simulink model "spi"  (Simulink 6.6)
settings: Solver=ode45  StartTime=0.0  StopTime=2000  RelTol=1e-3
libraries: xbsIndex_r4 x15, xps_library x1
settings Model: Creator=user  LastModifiedBy=SHL
settings GRTTargetCC: TargetFcnLib=ansi_tfl_table_tmw.mat

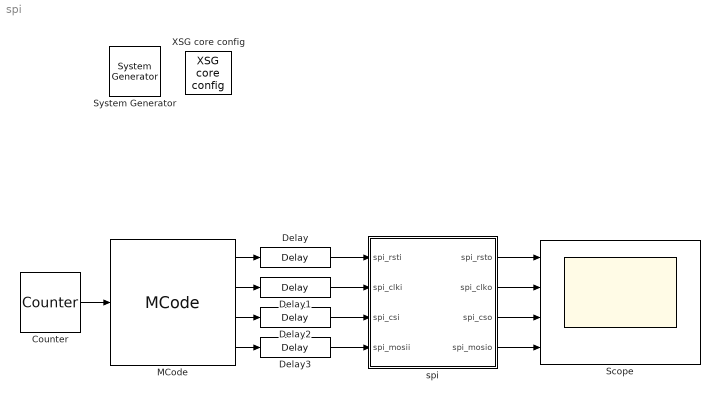
== system spi ==
  " System Generator" : xbsIndex_r4/ System Generator  Tag=genX  SystemSampleTime=-1  xilinxfamily=virtex5  part=xc5vsx95t  speed=-1  package=ff1136  synthesis_tool=XST  clock_wrapper=Clock Enables  directory=./spi/sysgen  testbench=off  simulink_period=1  sysclk_period=10  dcm_input_clock_period=100  incr_netlist=off  trim_vbits=Everywhere in SubSystem  dbl_ovrd=According to Block Masks  core_generation=According to Block Masks  run_coregen=off  deprecated_control=off  eval_field=0  block_type=sysgen
      settings: block_version=10.1.3
  Counter : xbsIndex_r4/Counter  cnt_type=Free Running  cnt_to=Inf  operation=Up  start_count=0  cnt_by_val=1  arith_type=Unsigned  n_bits=4  bin_pt=0  load_pin=off  rst=off  en=off  explicit_period=on  period=1  dbl_ovrd=off  use_behavioral_HDL=off  use_rpm=off  implementation=Fabric  block_type=counter
  Delay{,1..3} (4 alike) : xbsIndex_r4/Delay  en=off  latency=1  dbl_ovrd=off  reg_retiming=on  block_type=delay
  MCode : xbsIndex_r4/MCode  mfname=spi_ctrl  explicit_period=off  period=1  inputsTable={'boundInpExpr'=>[''],'inputs'=>['clk_in']}  outputsTable={'outputs'=>['spi_rst','spi_clk','spi_cs','spi_mosi'],'suppressOut'=>['off','off','off','off']}  dbl_ovrd=off  enable_stdout=off  enable_debug=off  suppress_output=1  defparams={}  hide_port_list={}  block_type=mcode
      settings: block_version=10.1.3
  Scope : Scope  NumInputPorts=4
      settings: TickLabels=on  YMin=-1~-1~-1~-1  YMax=2~2~2~2
  XSG core config : xps_library/XSG core config  Tag=xps:xsg  SystemSampleTime=-1  hw_sys=ROACH:sx95t  ibob_linux=off  clk_src=sys_clk  iBOB_clk_src=sys_clk  BEE2_ctrl_clk_src=sys_clk  BEE2_usr_clk_src=sys_clk  ROACH_clk_src=sys_clk  CORR_clk_src=sys_clk  gpio_clk_io_group=iBOB:sma  gpio_clk_bit_index=0  clk_rate=100  sample_period=1  synthesis_tool=XST  mpc_type=powerpc440_ext
  spi : Subsystem  Tag=xps:spi  AncestorBlock=xps_library/gpio
  wires:
  spi/3(spi_cso) -> Scope/3
  spi/4(spi_mosio) -> Scope/4
  Delay2/1 -> spi/3(spi_csi)
  Delay3/1 -> spi/4(spi_mosii)
  Counter/1 -> MCode/1
  MCode/1 -> Delay/1
  MCode/2 -> Delay1/1
  MCode/3 -> Delay2/1
  MCode/4 -> Delay3/1
  Delay/1 -> spi/1(spi_rsti)
  Delay1/1 -> spi/2(spi_clki)
  spi/1(spi_rsto) -> Scope/1
  spi/2(spi_clko) -> Scope/2

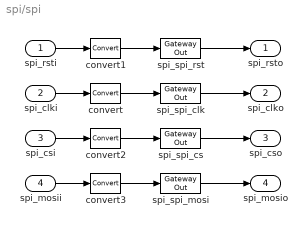
== system spi/spi ==
  spi_rsti : Inport
  spi_clki : Inport  Port=2
  spi_csi : Inport  Port=3
  spi_mosii : Inport  Port=4
  convert{,1..3} (4 alike) : xbsIndex_r4/Convert  arith_type=Boolean  n_bits=1  bin_pt=0  quantization=Truncate  overflow=Wrap  latency=0  dbl_ovrd=off  pipeline=off  block_type=convert
      settings: block_version=10.1.3
  spi_spi_clk : xbsIndex_r4/Gateway Out  hdl_port=on  timing_constraint=None  locs_specified=off  LOCs={}  block_type=gatewayout
      settings: infoedit="Gateway out block.  Converts Xilinx fixed point inputs into ouputs of type Simulink integer, double, or fixed point.<P><P>Hardware notes:  In hardware these blocks become top level output ports or are discarded, depending on how they are configured."  block_version=10.1.3
  spi_spi_cs : xbsIndex_r4/Gateway Out  hdl_port=on  timing_constraint=None  locs_specified=off  LOCs={}  block_type=gatewayout
      settings: infoedit="Gateway out block.  Converts Xilinx fixed point inputs into ouputs of type Simulink integer, double, or fixed point.<P><P>Hardware notes:  In hardware these blocks become top level output ports or are discarded, depending on how they are configured."  block_version=10.1.3
  spi_spi_mosi : xbsIndex_r4/Gateway Out  hdl_port=on  timing_constraint=None  locs_specified=off  LOCs={}  block_type=gatewayout
      settings: infoedit="Gateway out block.  Converts Xilinx fixed point inputs into ouputs of type Simulink integer, double, or fixed point.<P><P>Hardware notes:  In hardware these blocks become top level output ports or are discarded, depending on how they are configured."  block_version=10.1.3
  spi_spi_rst : xbsIndex_r4/Gateway Out  hdl_port=on  timing_constraint=None  locs_specified=off  LOCs={}  block_type=gatewayout
      settings: infoedit="Gateway out block.  Converts Xilinx fixed point inputs into ouputs of type Simulink integer, double, or fixed point.<P><P>Hardware notes:  In hardware these blocks become top level output ports or are discarded, depending on how they are configured."  block_version=10.1.3
  spi_rsto : Outport
  spi_clko : Outport  Port=2
  spi_cso : Outport  Port=3
  spi_mosio : Outport  Port=4
  wires:
  spi_clki/1 -> convert/1
  convert/1 -> spi_spi_clk/1
  spi_spi_clk/1 -> spi_clko/1
  spi_rsti/1 -> convert1/1
  convert1/1 -> spi_spi_rst/1
  spi_spi_rst/1 -> spi_rsto/1
  spi_csi/1 -> convert2/1
  convert2/1 -> spi_spi_cs/1
  spi_spi_cs/1 -> spi_cso/1
  spi_mosii/1 -> convert3/1
  convert3/1 -> spi_spi_mosi/1
  spi_spi_mosi/1 -> spi_mosio/1
